simulink model "test_plant"  (R2013a)
settings: Solver=ode45  StartTime=0.0  StopTime=10.0  MaxStep=1e-6  RelTol=1e-3
undefined symbols (not defined in the file or in its folder): Lc, Rc, Rsh
settings Model: Creator=mainster  LastModifiedBy=mainster

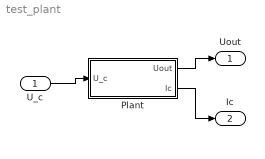
== system test_plant ==
  U_c : Inport
  Plant : Subsystem  Variant=on  OverrideUsingVariant=Variant_LR
  Uout : Outport
  Ic : Outport  Port=2
  wires:
  Plant/1(Uout) -> Uout/1
  Plant/2(Ic) -> Ic/1
  U_c/1 -> Plant/1(U_c)

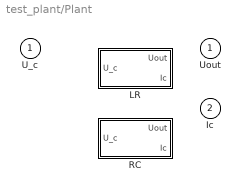
== system test_plant/Plant ==
  U_c : Inport
  LR : Subsystem  VariantControl=Variant_LR
  RC : Subsystem  VariantControl=Variant_RC
  Uout : Outport
  Ic : Outport  Port=2

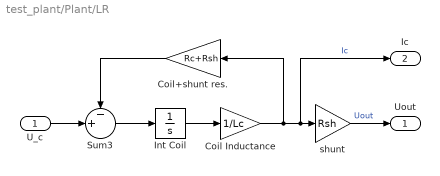
== system test_plant/Plant/LR ==
  U_c : Inport
  Coil Inductance : Gain  Gain=1/Lc
  Coil+shunt res. : Gain  Gain=Rc+Rsh
  Int Coil : Integrator
  Sum3 : Sum  Inputs=-+|
  shunt : Gain  Gain=Rsh
  Uout : Outport
  Ic : Outport  Port=2
  wires:
  U_c/1 -> Sum3/2
  Int Coil/1 -> Coil Inductance/1
  Coil+shunt res./1 -> Sum3/1
  Sum3/1 -> Int Coil/1
  Coil Inductance/1 -> Coil+shunt res./1, Ic/1, shunt/1  "Ic"
  shunt/1 -> Uout/1  "Uout"

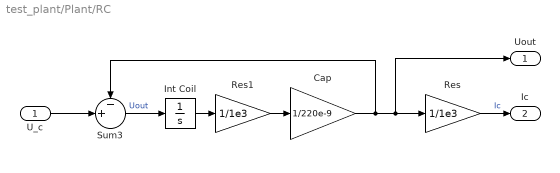
== system test_plant/Plant/RC ==
  U_c : Inport
  Cap : Gain  Gain=1/220e-9
  Int Coil : Integrator
  Res : Gain  Gain=1/1e3
  Res1 : Gain  Gain=1/1e3
  Sum3 : Sum  Inputs=-+|
  Uout : Outport
  Ic : Outport  Port=2
  wires:
  U_c/1 -> Sum3/2
  Sum3/1 -> Int Coil/1  "Uout"
  Res/1 -> Ic/1  "Ic"
  Cap/1 -> Sum3/1, Res/1, Uout/1
  Int Coil/1 -> Res1/1
  Res1/1 -> Cap/1
